simulink model "control_robot"  (R2018b)
settings: Solver=VariableStepAuto  StartTime=0.0  StopTime=40  FixedStep=1  RelTol=1e-3  EnableMultiTasking=on
PreLoadFcn:
  | sampleTime = 0.05;
  | 
  | % Vehicle Parameters
  | R = 0.1;
  | L = 0.5;
undefined symbols (not defined in the file or in its folder): DiscIntNeverNeededParam
libraries: mobileRoboticsLib x4, vrlib x1
settings Model: EnablePacing=on  Creator=scastro  LastModifiedBy=Toyin
settings DataIOCC: LimitDataPoints=on
settings OptimizationCC: LifeSpan=inf
settings DebuggingCC: AllowSymbolicDim=off  LibraryContextMissingDiagnostic=none  SFUnexpectedBacktrackingDiag=warning  SFNoUnconditionalDefaultTransitionDiag=warning  SFExecutionAtInitializationDiag=none
settings SFSimCC: SimUseLocalCustomCode=off
settings RTWCC: RTWUseLocalCustomCode=off
settings CodeAppCC: StateflowObjectComments=on
settings GRTTargetCC: TargetLangStandard=C89/C90 (ANSI)  GeneratePreprocessorConditionals=Disable all
settings ConfigComp: CovMetricSettings=dw  CovHtmlReporting=on  CovSaveCumulativeToWorkspaceVar=on  CovSaveSingleToWorkspaceVar=on  CovExternalEMLEnable=off  CovSFcnEnable=off
settings SimscapeCC: SimscapeNominalValues="[{\"value\":\"10\",\"unit\":\"V\"},{\"value\":\"1\",\"unit\":\"A\"},{\"value\":\"10\",\"unit\":\"N*m\"},{\"value\":\"10\",\"unit\":\"bar\"},{\"value\":\"100\",\"unit\":\"kJ/kg\"},{\"value\":\"1\",\"unit\":\"kW\"},{\"value\":\"300\",\"unit\":\"K\"},{\"value\":\"100\",\"unit\":\"cm^3/s\"},{\"value\":\"1\",\"unit\":\"kN\"},{\"value\":\"1\",\"unit\":\"g/cm^3\"},{\"value\":\"1\",\"unit\":\"l\"},{\"value\":\"1\",\"unit\":\"cm^2\"},{\"value\":\"60\",\"unit\":\"Hz\"}]"  SimscapeLogType=all  SimscapeLogDataHistory=10000
settings ConfigurationSet: Description=SimMechanics 2G
settings ExplorerConfigSet: InternalSimMechanicsExplorerSettings="<ExplorerConfiguration><canonicalview>default</canonicalview><AnimationSetting><BasePlaybackSpeed>1.0</BasePlaybackSpeed><PlaybackSpeedFactor>1.0</PlaybackSpeedFactor></AnimationSetting><TilePanel><TileInfo><Tiles Columns=\"1\" Count=\"1\" Rows=\"1\"><Column Weight=\"1\"/><Row Weight=\"1\"/><Tile Height=\"1\" Width=\"1\" X=\"0\" Y=\"0\"/></Tiles></TileInfo><SceneInfo><SceneViewer><BGColor><R>0.60000002384185791</R><G>0.60000002384185791</G><B>0.60000002384185791</B></BGColor><Camera><DoPerspective>off</DoPerspective><Position><X>-1.70656042355848525</X><Y>-0.974920623359631922</Y><Z>4.72930454537082046</Z></Position><Center><X>0.552860638431633689</X><Y>1.42025063411503494</Y><Z>1.4843509506914252</Z></Center><Up><X>0.664249622453917166</X><Y>0.300615402055903091</Y><Z>0.684399604848363485</Z></Up><ViewLimDist>1</ViewLimDist><YLim>2.77881717169207398</YLim><XLim>3.55928742670435394</XLim></Camera></SceneViewer></SceneInfo></TilePanel><MechEditorPanel><Cameras/><GfxPanelCameraMap/><VideoCreator><PlaybackSpeedRatio>1.0</PlaybackSpeedRatio><FrameRate>30</FrameRate><VideoFormat>Motion JPEG AVI</VideoFormat><FrameSize>auto</FrameSize></VideoCreator></MechEditorPanel></ExplorerConfiguration>"

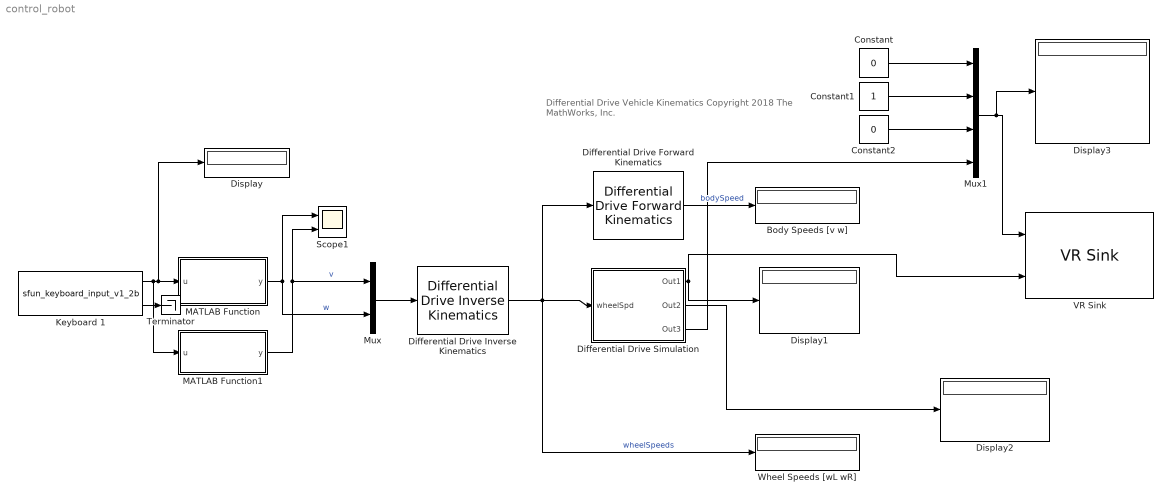
== system control_robot ==
  note: Differential Drive Vehicle Kinematics
      |
      | Copyright 2018 The MathWorks, Inc.
  Body Speeds [v w] : Display
  Constant : Constant  Value=0
  Constant1 : Constant
  Constant2 : Constant  Value=0
  Differential Drive Forward Kinematics : mobileRoboticsLib/Kinematic Models/Differential Drive/Differential Drive Forward Kinematics  wheelRadius=R  wheelBase=L
      settings: SourceProductName=Mobile Robotics Simulation Library
  Differential Drive Inverse Kinematics : mobileRoboticsLib/Kinematic Models/Differential Drive/Differential Drive Inverse Kinematics  wheelRadius=R  wheelBase=L
      settings: SourceProductName=Mobile Robotics Simulation Library
  Differential Drive Simulation : Subsystem  AncestorBlock=mobileRoboticsLib/Kinematic Models/Differential Drive/Differential Drive Simulation  mask(Differential Drive Simulation){wheelRadius=R, wheelBase=L, initX=0, initY=0, initAngle=0, Ts=sampleTime}
      mask prompts: wheelRadius "Wheel Radius [m]"; wheelBase "Wheelbase [m]"; initX "Initial X Position [m]"; initY "Initial Y Position [m]"; initAngle "Initial Angle [rad]"; Ts "Sample Time"
      mask help:
      | Simulates the kinematics of a differential drive vehicle from a specified initial pose.
      |
      | Input: Left and right wheel speeds [wL; wR], in rad/s
      |
      | Output: Pose [x; y; theta], in m, m, and rad
      |
      | Set the Sample Time parameter to 0 for continuous-time simulation, or a positive number for discrete-time simulation.
      mask Help: web('matlab:edit mrsDocDifferentialDrive')
  Display{,1..3} (4 alike) : Display
  Keyboard 1 : M-S-Function  FunctionName=sfun_keyboard_input_v1_2b  mask(Keyboard Input){}
      mask help: Keyboard Input
      mask Display: fprintf('Keyboard');
  MATLAB Function : MATLAB Function  TreatAsAtomicUnit=on
  MATLAB Function1 : MATLAB Function  TreatAsAtomicUnit=on
  Mux : Mux  Inputs=2
  Mux1 : Mux
  Scope1 : Scope  NumInputPorts=2
  Terminator : Terminator
  VR Sink : vrlib/VR Sink  InstantiateOnLoad=on  SampleTime=0.1  ViewEnable=on  RemoteChange=off  RemoteView=off  FieldsWritten=Chair_Wheels.rotation.4.1.1.double#Chair_Wheels.translation.3.1.1.double  WorldFileName=wheelchair_wheels.wrl  AutoView=off  VideoDimensions=[]  AllowVariableSize=off
      settings: SourceProductBaseCode=VR
  Wheel Speeds [wL wR] : Display
  wires:
  Differential Drive Inverse Kinematics/1 -> Differential Drive Simulation/1(wheelSpd), Differential Drive Forward Kinematics/1, Wheel Speeds [wL wR]/1  "wheelSpeeds"
  Mux/1 -> Differential Drive Inverse Kinematics/1
  Differential Drive Forward Kinematics/1 -> Body Speeds [v w]/1  "bodySpeed"
  Keyboard 1/1 -> MATLAB Function1/1(u), Display/1, MATLAB Function/1(u)
  Keyboard 1/2 -> Terminator/1
  MATLAB Function/1(y) -> Mux/2, Scope1/1  "w"
  MATLAB Function1/1(y) -> Mux/1, Scope1/2  "v"
  Differential Drive Simulation/1(Out1) -> Display1/1, VR Sink/2
  Differential Drive Simulation/2(Out2) -> Display2/1
  Differential Drive Simulation/3(Out3) -> Mux1/4
  Mux1/1 -> Display3/1, VR Sink/1
  Constant/1 -> Mux1/1
  Constant1/1 -> Mux1/2
  Constant2/1 -> Mux1/3

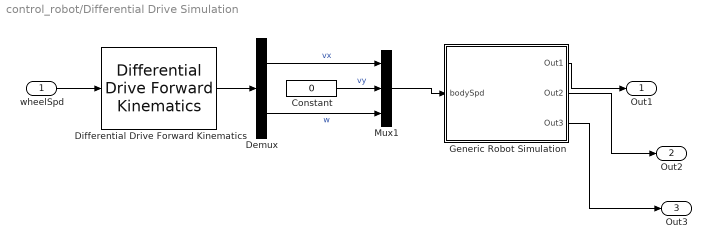
== system control_robot/Differential Drive Simulation ==
  wheelSpd : Inport
  Constant : Constant  Value=0
  Demux : Demux  Outputs=2
  Differential Drive Forward Kinematics : mobileRoboticsLib/Kinematic Models/Differential Drive/Differential Drive Forward Kinematics  wheelRadius=wheelRadius  wheelBase=wheelBase
      settings: SourceProductName=Mobile Robotics Simulation Toolbox
  Generic Robot Simulation : Subsystem  AncestorBlock=mobileRoboticsLib/Utilities/Generic Vehicle Simulation  mask(Generic Vehicle Simulation){initX=initX, initY=initY, initAngle=initAngle, Ts=Ts}
      mask prompts: initX "Initial X Position [m]"; initY "Initial Y Position [m]"; initAngle "Initial Angle (theta) [rad]"; Ts "Sample Time"
      mask help:
      | Simulates the kinematics of a generic vehicle, from a specified initial pose.
      |
      | Input: Body velocities [vx; vy; w], in m/s, m/s, and rad/s
      |
      | Output: Pose [x; y; theta], in m, m, and rad
      |
      | Set the Sample Time parameter to 0 for continuous-time simulation, or a positive number for discrete-time simulation.
      mask init:
      | blk = [gcb '/Velocity Integrator'];
      | if Ts > 0
      |     set_param(blk,'OverrideUsingVariant','mode==2');  
      | else
      |     set_param(blk,'OverrideUsingVariant','mode==1');  
      | end
  Mux1 : Mux  Inputs=3
  Out1 : Outport
  Out2 : Outport  Port=2
  Out3 : Outport  Port=3
  wires:
  Differential Drive Forward Kinematics/1 -> Demux/1
  wheelSpd/1 -> Differential Drive Forward Kinematics/1
  Constant/1 -> Mux1/2  "vy"
  Demux/2 -> Mux1/3  "w"
  Demux/1 -> Mux1/1  "vx"
  Mux1/1 -> Generic Robot Simulation/1(bodySpd)
  Generic Robot Simulation/1(Out1) -> Out1/1
  Generic Robot Simulation/2(Out2) -> Out2/1
  Generic Robot Simulation/3(Out3) -> Out3/1

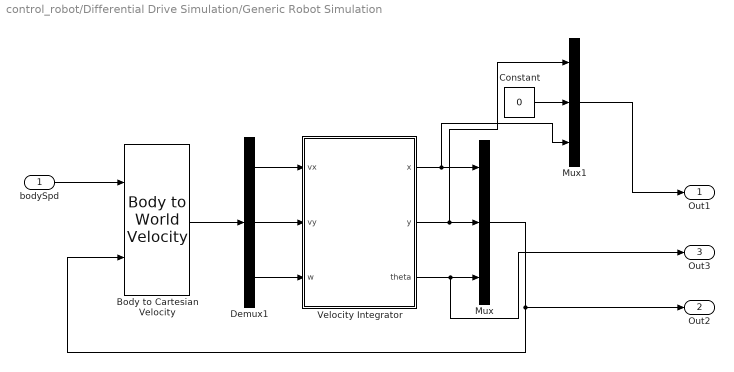
== system control_robot/Differential Drive Simulation/Generic Robot Simulation ==
  bodySpd : Inport
  Body to Cartesian Velocity : mobileRoboticsLib/Utilities/Body to World Velocity
      settings: SourceProductName=Mobile Robotics Simulation Toolbox
  Constant : Constant  Value=0
  Demux1 : Demux  Outputs=3
  Mux : Mux  Inputs=3
  Mux1 : Mux  Inputs=3
  Velocity Integrator : Subsystem  VariantControlMode=Label  Variant=on  VariantControl=Variant1  LabelModeActiveChoice=mode==2
  Out1 : Outport
  Out2 : Outport  Port=2
  Out3 : Outport  Port=3
  wires:
  Velocity Integrator/3(" theta") -> Out3/1, Mux/3
  Velocity Integrator/2(" y") -> Mux1/1, Mux/2
  Velocity Integrator/1(" x") -> Mux1/3, Mux/1
  Mux/1 -> Out2/1, Body to Cartesian Velocity/2
  Body to Cartesian Velocity/1 -> Demux1/1
  Demux1/1 -> Velocity Integrator/1("vx ")
  Demux1/2 -> Velocity Integrator/2("vy ")
  Demux1/3 -> Velocity Integrator/3("w ")
  bodySpd/1 -> Body to Cartesian Velocity/1
  Mux1/1 -> Out1/1
  Constant/1 -> Mux1/2

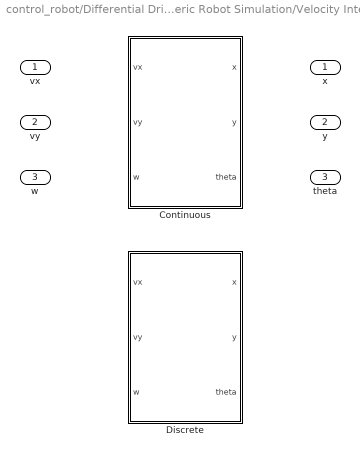
== system control_robot/Differential Drive Simulation/Generic Robot Simulation/Velocity Integrator ==
  "vx " : Inport
  "vy " : Inport  Port=2
  "w " : Inport  Port=3
  Continuous : Subsystem  VariantControl=mode==1
  Discrete : Subsystem  VariantControl=mode==2
  " x" : Outport
  " y" : Outport  Port=2
  " theta" : Outport  Port=3

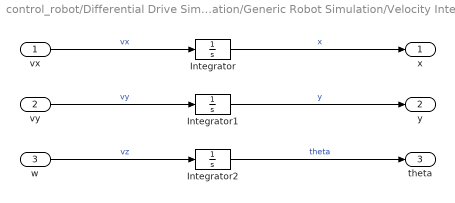
== system control_robot/Differential Drive Simulation/Generic Robot Simulation/Velocity Integrator/Continuous ==
  vx : Inport
  vy : Inport  Port=2
  w : Inport  Port=3
  Integrator : Integrator  InitialCondition=initX
  Integrator1 : Integrator  InitialCondition=initY
  Integrator2 : Integrator  InitialCondition=initAngle
  x : Outport
  y : Outport  Port=2
  theta : Outport  Port=3
  wires:
  Integrator2/1 -> theta/1  "theta"
  w/1 -> Integrator2/1  "vz"
  vx/1 -> Integrator/1  "vx"
  Integrator/1 -> x/1  "x"
  vy/1 -> Integrator1/1  "vy"
  Integrator1/1 -> y/1  "y"

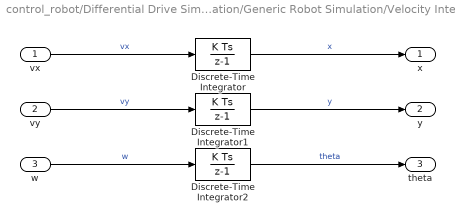
== system control_robot/Differential Drive Simulation/Generic Robot Simulation/Velocity Integrator/Discrete ==
  vx : Inport
  vy : Inport  Port=2
  w : Inport  Port=3
  Discrete-Time Integrator : DiscreteIntegrator  InitialCondition=initX  SampleTime=Ts  ICPrevOutput=DiscIntNeverNeededParam  ICPrevScaledInput=DiscIntNeverNeededParam
  Discrete-Time Integrator1 : DiscreteIntegrator  InitialCondition=initY  SampleTime=Ts  ICPrevOutput=DiscIntNeverNeededParam  ICPrevScaledInput=DiscIntNeverNeededParam
  Discrete-Time Integrator2 : DiscreteIntegrator  InitialCondition=initAngle  SampleTime=Ts  ICPrevOutput=DiscIntNeverNeededParam  ICPrevScaledInput=DiscIntNeverNeededParam
  x : Outport
  y : Outport  Port=2
  theta : Outport  Port=3
  wires:
  Discrete-Time Integrator1/1 -> y/1  "y"
  vy/1 -> Discrete-Time Integrator1/1  "vy"
  Discrete-Time Integrator/1 -> x/1  "x"
  vx/1 -> Discrete-Time Integrator/1  "vx"
  w/1 -> Discrete-Time Integrator2/1  "w"
  Discrete-Time Integrator2/1 -> theta/1  "theta"

== matlab function control_robot/MATLAB Function ==
  data: u input; y output
function y = angular_velocity(u)
if u == 30 %forward
    y = 0;
% elseif u == 49 %decrease speed
%     y = 0;
% elseif u == 50 %increase speed
%     y = 0;
elseif u == 28 %left
    y = pi;
elseif u == 29 %right
    y = -pi;
elseif u == 31 %backward
    y = 0;
else
    y = 0;
end
end

== matlab function control_robot/MATLAB Function1 ==
  data: u input; y output
function y = linear_velocity(u)
if u == 30 %forward
    y = 2;
% elseif u == 49 %decrease speed
%     y = 1;
% elseif u == 50 %increase speed
%     y = 3;
elseif u == 28 %left
    y = 1;
elseif u == 29 %right 
    y = 1;
elseif u == 31 %backward
    y = -1;
else
    y = 0;
end
end
